simulink model "EOR_CSTmod"  (R2020b)
settings: Solver=FixedStepAuto  StartTime=0.0  StopTime=TMax  FixedStep=DT  RelTol=1e-3  EnableMultiTasking=on
values from neighbouring files (symbols this model uses):
  M_rated = 1e-6 * P_rated / Omega_rated    [EOR_CSTmod_init.m]    (also in EOR_init.m)
  windspeed = simin.getVariable('windspeed')    [EOR_CSTmod_init.m]
undefined symbols (not defined in the file or in its folder): BLCTRL_M_2, BLCTRL_theta_max, BLCTRL_theta_rate, BLCTRL_theta_star, BLCTRL_torque_rate, EOR_A2, EOR_A3, EOR_B2, EOR_B3, EOR_C2e, EOR_C3e, EOR_D2eu, EOR_D2ew, EOR_D3eu, EOR_D3ew, EOR_E2w, EOR_E3w, EOR_F2, EOR_F3, EOR_filt_a, EOR_filt_b, EOR_T, EOR_T_setup, EOR_T_solve, EOR_u_star, EOR_x_star
libraries: ctrlSharedLib x1
settings Model: Creator=lpwoolcock  LastModifiedBy=lpwoolcock

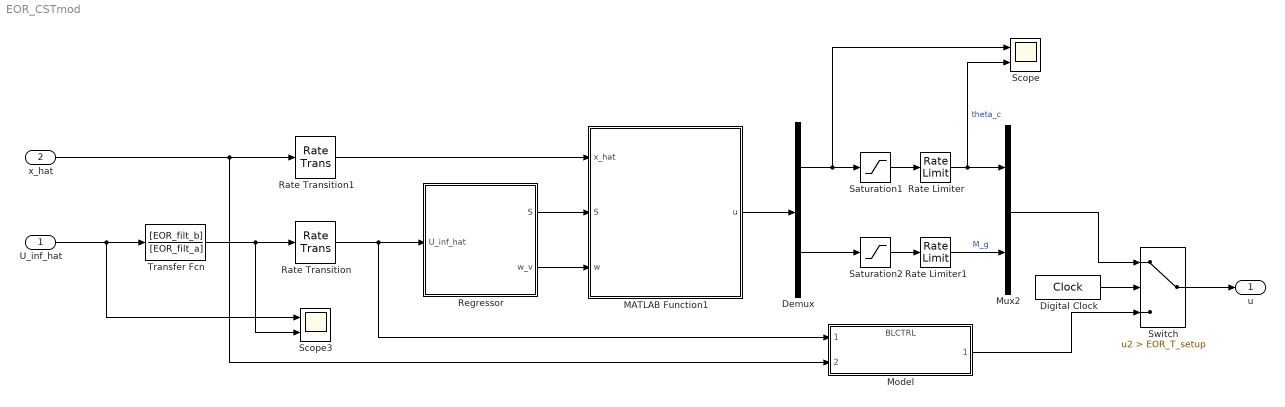
== system EOR_CSTmod ==
  U_inf_hat : Inport  PortDimensions=1
  x_hat : Inport  Port=2  PortDimensions=[5 1]
  Demux : Demux  Outputs=2
  Digital Clock : DigitalClock  SampleTime=EOR_T
  MATLAB Function1 : MATLAB Function  TreatAsAtomicUnit=on
  Model : ModelReference  ModelNameDialog=BLCTRL.slx  SimulationMode=Normal  ModelReferenceVersion=2.4
  Mux2 : Mux  Inputs=2
  Rate Limiter : RateLimiter  RisingSlewLimit=BLCTRL_theta_rate  FallingSlewLimit=-BLCTRL_theta_rate  SampleTimeMode=inherited
  Rate Limiter1 : RateLimiter  RisingSlewLimit=BLCTRL_torque_rate  FallingSlewLimit=-BLCTRL_torque_rate  SampleTimeMode=inherited
  Rate Transition : RateTransition  OutPortSampleTime=EOR_T
  Rate Transition1 : RateTransition  InitialCondition=zeros(5,1)  OutPortSampleTime=EOR_T
  Regressor : Subsystem
  Saturation1 : Saturate  UpperLimit=BLCTRL_theta_max  LowerLimit=BLCTRL_theta_star
  Saturation2 : Saturate  UpperLimit=1.1*BLCTRL_M_2  LowerLimit=-1.1*BLCTRL_M_2
  Scope : Scope  NumInputPorts=2
  Scope3 : Scope  NumInputPorts=2
  Switch : Switch  Criteria=u2 > Threshold  Threshold=EOR_T_setup
  Transfer Fcn : TransferFcn  Numerator=[EOR_filt_b]  Denominator=[EOR_filt_a]
  u : Outport  PortDimensions=[2 1]
  wires:
  Switch/1 -> u/1
  x_hat/1 -> Model/2, Rate Transition1/1
  Regressor/1(S) -> MATLAB Function1/2(S)
  Mux2/1 -> Switch/1
  Model/1 -> Switch/3
  Digital Clock/1 -> Switch/2
  Regressor/2(w_v) -> MATLAB Function1/3(w)
  Rate Transition/1 -> Regressor/1(U_inf_hat), Model/1
  Transfer Fcn/1 -> Scope3/2, Rate Transition/1
  U_inf_hat/1 -> Scope3/1, Transfer Fcn/1
  Saturation1/1 -> Rate Limiter/1
  Saturation2/1 -> Rate Limiter1/1
  Rate Limiter1/1 -> Mux2/2  "M_g"
  Rate Limiter/1 -> Scope/2, Mux2/1  "theta_c"
  Rate Transition1/1 -> MATLAB Function1/1(x_hat)
  Demux/1 -> Scope/1, Saturation1/1
  MATLAB Function1/1(u) -> Demux/1
  Demux/2 -> Saturation2/1

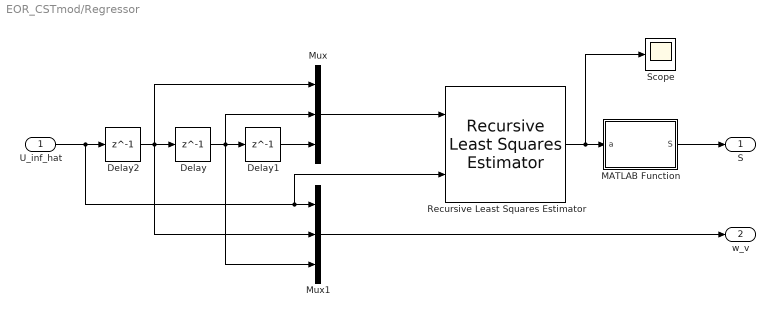
== system EOR_CSTmod/Regressor ==
  U_inf_hat : Inport
  Delay : Delay  DelayLength=1
  Delay1 : Delay  DelayLength=1
  Delay2 : Delay  DelayLength=1
  MATLAB Function : MATLAB Function  TreatAsAtomicUnit=on
  Mux : Mux  Inputs=3
  Mux1 : Mux  Inputs=3
  Recursive Least Squares Estimator : ctrlSharedLib/Recursive Least Squares Estimator  InitialEstimateSource=None  InitialParameterData=3  P0=1e4  InitialRegressors=0  InitialOutputs=0  History=Infinite  WindowLength=200  EstimationMethod=Forgetting Factor  AdaptationParameter=0.99  HasTimeVaryingAdaptationParameter=off  NormalizationBias=eps  OutputError=off  OutputP=off  AddEnablePort=off  InputProcessing=Sample-based  Ts=EOR_T
      settings: SourceProductBaseCode=CT,ID
  Scope : Scope
  S : Outport
  w_v : Outport  Port=2
  wires:
  Delay/1 -> Mux1/3, Mux/2, Delay1/1
  Delay1/1 -> Mux/3
  Delay2/1 -> Mux1/2, Mux/1, Delay/1
  U_inf_hat/1 -> Recursive Least Squares Estimator/2, Mux1/1, Delay2/1
  Mux/1 -> Recursive Least Squares Estimator/1
  Mux1/1 -> w_v/1
  Recursive Least Squares Estimator/1 -> Scope/1, MATLAB Function/1(a)
  MATLAB Function/1(S) -> S/1

== matlab function EOR_CSTmod/Regressor/MATLAB Function ==
  data: a input; S output size=[3 3]
function S = fcn(a)

    S = [a(1) a(2) a(3); 1 0 0; 0 1 0];

end

== matlab function EOR_CSTmod/MATLAB Function1 ==
  data: x_hat input size=[5 1]; u output size=[2 1]; S input size=[3 3]; w input size=[3 1]; EOR_T parameter size=1; EOR_T_solve parameter size=1; EOR_x_star parameter size=[5 1]; EOR_A2 parameter size=[3 3]; EOR_B2 parameter size=[3 1]; EOR_C2e parameter size=[1 3]; EOR_u_star parameter size=[2 1]; EOR_E2w parameter size=[3 3]; EOR_D2eu parameter size=1; EOR_D2ew parameter size=[1 3]; EOR_A3 parameter size=[2 2]; EOR_B3 parameter size=[2 1]; EOR_C3e parameter size=[1 2]; EOR_E3w parameter size=[2 3]; EOR_D3eu parameter size=1; EOR_D3ew parameter size=[1 3]; windspeed parameter size=1; EOR_F3 parameter size=[1 2]; EOR_F2 parameter size=[1 3]; M_rated parameter size=1
function u  = EOR(x_hat, S, w, EOR_T, EOR_T_solve, EOR_x_star, EOR_A2, EOR_B2, EOR_C2e, EOR_u_star, EOR_E2w, EOR_D2eu, EOR_D2ew, EOR_A3, EOR_B3, EOR_C3e, EOR_E3w, EOR_D3eu, EOR_D3ew, windspeed, EOR_F3, EOR_F2, M_rated)

    persistent t;
    if isempty(t)
        t = 0;
    end
    
    persistent G2 G3;
    if isempty(G2)
        G2 = zeros(1,3);
        G3 = zeros(1,3);
    end
    
    if t >= EOR_T_solve
        

        Gamma2 = zeros(1,3);
        Pi2 = zeros(3,3);

        [Pi2, Gamma2] = EOR_solve(EOR_A2, EOR_B2, EOR_E2w, EOR_C2e, EOR_D2eu, EOR_D2ew, S);
        G2 = Gamma2 - EOR_F2 * Pi2;

        Gamma3 = zeros(1,3);
        Pi3 = zeros(2,3);

        [Pi3, Gamma3] = EOR_solve(EOR_A3, EOR_B3, EOR_E3w, EOR_C3e, EOR_D3eu, EOR_D3ew, S);
        G3 = Gamma3 - EOR_F3 * Pi3;


        t = 0;
    end
    

    
    theta_c = EOR_u_star(1) + EOR_F3 * (x_hat(4:5) - EOR_x_star(4:5)) + G3 * (w - windspeed);
    
    M_g = EOR_u_star(2) + EOR_F2 * (x_hat(1:3) - EOR_x_star(1:3)) + G2 * (w - windspeed);
    
    if theta_c < 0
        theta_c = 0;
    elseif theta_c > pi/180
        M_g = M_rated;
    end
    
   % u = zeros(2,1);
    
    u = [theta_c; M_g];    
    t = t + EOR_T;
end
